simulink model "C172S_IntegratedAutopilot_V1"  (R2026a)
settings: Solver=ode4  StartTime=0  StopTime=180  FixedStep=0.01
InitFcn:
  | ah1Data = c172sLongitudinalData();
  | [~,ah1Plant] = c172sLongitudinalPlant(ah1Data);
  | ah1PitchController = c172sPitchAttitudeControllerData();
  | ah1Actuator = c172sElevatorActuatorData();
  | ah1AltitudeController = c172sAltitudeHoldControllerData();
  | A_ah1 = ah1Plant.A; B_ah1 = ah1Plant.B;
  | C_ah1 = ah1Plant.C; D_ah1 = ah1Plant.D;
  | Vtrim_ah1_mps = ah1Data.trim.V_mps;
  | Kh_ah1_per_s = ah1AltitudeController.altitudeGain_per_s;
  | Kv_ah1_radPerMps = ah1AltitudeController.verticalSpeedGain_radPerMps;
  | tauAltitude_ah1_s = ah1AltitudeController.commandFilterTimeConstant_s;
  | hDotLimit_ah1_mps = ah1AltitudeController.verticalSpeedCommandLimit_mps;
  | thetaLimit_ah1_rad = ah1AltitudeController.pitchCommandLimit_rad;
  | Kp_ah1 = ah1PitchController.Kp_radPerRad;
  | Ki_ah1_per_s = ah1PitchController.Ki_radPerRadPerS;
  | Kq_ah1_s = ah1Actuator.integration.Kq_s;
  | tauTheta_ah1_s = ah1PitchController.commandFilterTimeConstant_s;
  | tauActuator_ah1_s = ah1Actuator.dynamics.timeConstant_s;
  | Tt_ah1_s = ah1Actuator.antiWindup.trackingTimeConstant_s;
  | deltaELower_ah1_rad = ah1Actuator.authority.lowerLimit_rad;
  | deltaEUpper_ah1_rad = ah1Actuator.authority.upperLimit_rad;
  | deltaERate_ah1_radps = deg2rad(ah1Actuator.dynamics.rateLimit_degps);
  | if ~exist('hCommand_ah1_m','var'), hCommand_ah1_m = ah1AltitudeController.validation.operationalCommand_m; end
  | if ~exist('antiWindupEnable_ah1','var'), antiWindupEnable_ah1 = 1.0; end
  | if ~exist('x0_ah1','var'), x0_ah1 = zeros(4,1); end
  | if ~exist('xi0_ah1','var'), xi0_ah1 = 0.0; end
  | if ~exist('deltaE0_ah1','var'), deltaE0_ah1 = 0.0; end
  | if ~exist('h0_ah1_m','var'), h0_ah1_m = 0.0; end
  | hh1Data = c172sLateralDirectionalData();
  | [~,hh1Plant] = c172sLateralDirectionalPlant(hh1Data);
  | hh1YawController = c172sYawDamperData();
  | hh1RudderActuator = c172sRudderActuatorData();
  | hh1RollController = c172sRollAttitudeControllerData();
  | hh1AileronActuator = c172sAileronActuatorData();
  | hh1HeadingSensor = c172sHeadingSensorData();
  | hh1HeadingController = c172sHeadingHoldControllerData();
  | if ~strcmp(hh1Data.model.version,hh1HeadingController.requiredPlantVersion), error('HH V1 plant dependency mismatch.'); end
  | if ~strcmp(hh1YawController.artifactRevision,hh1HeadingController.requiredYawDamperRevision), error('HH V1 yaw-controller dependency mismatch.'); end
  | if ~strcmp(hh1RudderActuator.artifactRevision,hh1HeadingController.requiredRudderAuditRevision), error('HH V1 rudder-audit dependency mismatch.'); end
  | if ~strcmp(hh1AileronActuator.artifactRevision,hh1HeadingController.requiredAileronAuditRevision), error('HH V1 aileron-audit dependency mismatch.'); end
  | if ~strcmp(hh1RollController.artifactRevision,hh1HeadingController.requiredRollControllerRevision), error('HH V1 roll-controller dependency mismatch.'); end
  | if ~strcmp(hh1HeadingSensor.artifactRevision,hh1HeadingController.requiredHeadingSensorRevision), error('HH V1 heading-sensor dependency mismatch.'); end
  | A_hh1 = hh1Plant.A; B_hh1 = hh1Plant.B;
  | C_hh1 = hh1Plant.C; D_hh1 = hh1Plant.D;
  | Kphi_hh1 = hh1RollController.bankProportionalGain;
  | Ki_hh1 = hh1RollController.bankIntegralGain_per_s;
  | Kp_hh1 = hh1RollController.rollRateGain_s;
  | Tcmd_hh1 = hh1RollController.commandFilterTimeConstant_s;
  | Kr_hh1 = hh1YawController.rudderGain_s;
  | Tw_hh1 = hh1YawController.washoutTimeConstant_s;
  | TsRudder_hh1 = hh1RudderActuator.sensor.filterTimeConstant_s;
  | tauRudder_hh1 = hh1RudderActuator.dynamics.timeConstant_s;
  | TsRoll_hh1 = hh1AileronActuator.sensor.filterTimeConstant_s;
  | tauAileron_hh1 = hh1AileronActuator.dynamics.timeConstant_s;
  | Tt_hh1 = hh1AileronActuator.antiWindup.trackingTimeConstant_s;
  | delaySampleTime_hh1 = hh1AileronActuator.sensor.nominalDelay_s;
  | Kpsi_hh1 = hh1HeadingController.headingErrorGain;
  | TsHeading_hh1 = hh1HeadingSensor.filterTimeConstant_s;
  | headingDelaySampleTime_hh1 = hh1HeadingSensor.nominalDelay_s/5;
  | bankCommandLower_hh1_rad = -deg2rad(hh1HeadingController.bankCommandAuthority_deg);
  | ... (+50 lines)
undefined symbols (not defined in the file or in its folder): aileronPulseEnd_hh1_s, aileronPulseStart_hh1_s, antiWindupEnable_ah1, antiWindupEnable_hh1, deltaAAuto0_hh1_rad, deltaE0_ah1, deltaRAuto0_hh1_rad, filteredCommand0_hh1_rad, h0_ah1_m, headingBias_hh1_rad, headingNoiseAmplitude_hh1_rad, headingNoiseFrequency_hh1_radps, pDelay0_hh1_radps, phiDelay0_hh1_rad, phiNoiseAmplitude_hh1_rad, phiNoiseFrequency_hh1_radps, phiSensor0_hh1_rad, pilotAileronBias_hh1_rad, pilotAileronPulse_hh1_rad, pilotRudderBias_hh1_rad, pilotRudderPulse_hh1_rad, pNoiseAmplitude_hh1_radps, pNoiseFrequency_hh1_radps, pSensor0_hh1_radps, psiDelay0_hh1_rad, psiSensor0_hh1_rad, rDelay0_hh1_radps, rSensor0_hh1_radps, rudderPulseEnd_hh1_s, rudderPulseStart_hh1_s, x0_ah1, x0_hh1, xi0_ah1, xi0_hh1_rad_s, xw0_hh1_radps, yawNoiseAmplitude_hh1_radps, yawNoiseFrequency_hh1_radps
(part 2 of 2)

== matlab function C172S_IntegratedAutopilot_V1/Frozen Executable Mode Manager V1/Independent Executable Mode Manager ==
  settings: updateMethod=DISCRETE  sampleTime=0.01
  data: engageRequest input; engaged output; disconnectRequest input; pilotOverride input; trimStable input; coreValid input; headingValid input; altitudeValid input; aileronSaturated input; elevatorSaturated input; lateralRequest input; verticalRequest input; updateHeading input; updateAltitude input; bank_deg input; pitch_deg input; heading_deg input; altitude_ft input; selectedHeading_deg input; selectedAltitude_ft input; lateralMode output; verticalMode output; rollEnable output; headingEnable output; pitchEnable output; altitudeEnable output; bankCommand_deg output; pitchCommand_deg output; headingCommand_deg output; altitudeCommand_ft output; rollTrack output; pitchTrack output; disconnectTone output; eventCode output; coreTimer_s output; headingTimer_s output; altitudeTimer_s output; aileronSatTimer_s output; elevatorSatTimer_s output
function [engaged,lateralMode,verticalMode,rollEnable,headingEnable,pitchEnable,altitudeEnable,bankCommand_deg,pitchCommand_deg,headingCommand_deg,altitudeCommand_ft,rollTrack,pitchTrack,disconnectTone,eventCode,coreTimer_s,headingTimer_s,altitudeTimer_s,aileronSatTimer_s,elevatorSatTimer_s] = supervisor(engageRequest,disconnectRequest,pilotOverride,trimStable,coreValid,headingValid,altitudeValid,aileronSaturated,elevatorSaturated,lateralRequest,verticalRequest,updateHeading,updateAltitude,bank_deg,pitch_deg,heading_deg,altitude_ft,selectedHeading_deg,selectedAltitude_ft)
%#codegen
persistent ap lat vert bankRef pitchRef headingRef altitudeRef
persistent coreTimer headingTimer altitudeTimer aileronTimer elevatorTimer
if isempty(ap)
    ap = false; lat = 0; vert = 0;
    bankRef = captureBank(bank_deg); pitchRef = capturePitch(pitch_deg);
    headingRef = normalizeHeading(heading_deg); altitudeRef = altitude_ft;
    coreTimer = 0.0; headingTimer = 0.0; altitudeTimer = 0.0;
    aileronTimer = 0.0; elevatorTimer = 0.0;
end
dt = 0.01;
eventCode = 0; rollTrack = 0; pitchTrack = 0; disconnectTone = 0;
wasEngaged = ap;
coreTimer = timerUpdate(coreValid < 0.5,coreTimer,dt);
headingTimer = timerUpdate(headingValid < 0.5,headingTimer,dt);
altitudeTimer = timerUpdate(altitudeValid < 0.5,altitudeTimer,dt);
aileronTimer = timerUpdate(aileronSaturated > 0.5,aileronTimer,dt);
elevatorTimer = timerUpdate(elevatorSaturated > 0.5,elevatorTimer,dt);
if ap
    if disconnectRequest > 0.5
        ap = false; lat = 0; vert = 0; eventCode = 7; disconnectTone = 1;
    elseif pilotOverride > 0.5
        ap = false; lat = 0; vert = 0; eventCode = 8; disconnectTone = 1;
    elseif abs(bank_deg) > 30 || abs(pitch_deg) > 10
        ap = false; lat = 0; vert = 0; eventCode = 11; disconnectTone = 1;
    elseif coreTimer + 1.0e-12 >= 0.10000000000000001
        ap = false; lat = 0; vert = 0; eventCode = 9; disconnectTone = 1;
    elseif max(aileronTimer,elevatorTimer) + 1.0e-12 >= 2
        ap = false; lat = 0; vert = 0; eventCode = 10; disconnectTone = 1;
    end
end
if ~ap
    if ~wasEngaged && engageRequest > 0.5
        permitted = trimStable > 0.5 && coreValid > 0.5 && pilotOverride < 0.5 && aileronSaturated < 0.5 && elevatorSaturated < 0.5;
        if lateralRequest == 2, permitted = permitted && headingValid > 0.5; end
        if verticalRequest == 2, permitted = permitted && altitudeValid > 0.5; end
        if permitted
            ap = true; eventCode = 1; rollTrack = 1; pitchTrack = 1;
            if lateralRequest == 2
                lat = 2; headingRef = normalizeHeading(selectedHeading_deg);
            else
                lat = 1; bankRef = captureBank(bank_deg);
            end
            if verticalRequest == 2
                vert = 2; altitudeRef = selectedAltitude_ft;
            else
                vert = 1; pitchRef = capturePitch(pitch_deg);
            end
        else
            eventCode = 4;
        end
    end
else
    if lat == 2 && headingTimer + 1.0e-12 >= 0.10000000000000001
        lat = 1; bankRef = captureBank(bank_deg); rollTrack = 1; eventCode = 5;
    end
    if vert == 2 && altitudeTimer + 1.0e-12 >= 0.10000000000000001
        vert = 1; pitchRef = capturePitch(pitch_deg); pitchTrack = 1; eventCode = 6;
    end
    if lateralRequest ~= 0
        if lateralRequest == 1
            lat = 1; bankRef = captureBank(bank_deg); rollTrack = 1; eventCode = 2;
        elseif lateralRequest == 2 && headingValid > 0.5
            lat = 2; headingRef = normalizeHeading(selectedHeading_deg); rollTrack = 1; eventCode = 2;
        else
            eventCode = 3;
        end
    end
    if verticalRequest ~= 0
        if verticalRequest == 1
            vert = 1; pitchRef = capturePitch(pitch_deg); pitchTrack = 1; eventCode = 2;
        elseif verticalRequest == 2 && altitudeValid > 0.5
            vert = 2; altitudeRef = selectedAltitude_ft; pitchTrack = 1; eventCode = 2;
        else
            eventCode = 3;
        end
    end
    if lat == 2 && updateHeading > 0.5 && headingValid > 0.5
        headingRef = normalizeHeading(selectedHeading_deg);
    end
    if vert == 2 && updateAltitude > 0.5 && altitudeValid > 0.5
        altitudeRef = selectedAltitude_ft;
    end
end
engaged = double(ap); lateralMode = lat; verticalMode = vert;
rollEnable = double(ap && lat == 1); headingEnable = double(ap && lat == 2);
pitchEnable = double(ap && vert == 1); altitudeEnable = double(ap && vert == 2);
bankCommand_deg = 0.0; pitchCommand_deg = 0.0;
if ap && lat == 1, bankCommand_deg = bankRef; end
if ap && vert == 1, pitchCommand_deg = pitchRef; end
headingCommand_deg = headingRef; altitudeCommand_ft = altitudeRef;
coreTimer_s = coreTimer; headingTimer_s = headingTimer; altitudeTimer_s = altitudeTimer;
aileronSatTimer_s = aileronTimer; elevatorSatTimer_s = elevatorTimer;
end
function value = captureBank(value)
if abs(value) < 6
    value = 0.0;
else
    value = min(max(value,-20),20);
end
end
function value = capturePitch(value)
value = min(max(value,-3),3);
end
function value = normalizeHeading(value)
value = mod(value,360.0);
if value < 0.0, value = value + 360.0; end
end
function timer = timerUpdate(condition,timer,dt)
if condition, timer = timer + dt; else, timer = 0.0; end
end
